simulink model "adaptive"  (R2020a)
settings: Solver=VariableStepAuto  StartTime=0.0  StopTime=30.0  RelTol=1e-3
values from neighbouring files (symbols this model uses):
  Ts = 0.1    [main_adaptive_mpc.m]
libraries: simulink x2, mpclib x1, cstblocks x1
settings Model: Creator=lamarre  LastModifiedBy=Lamarre

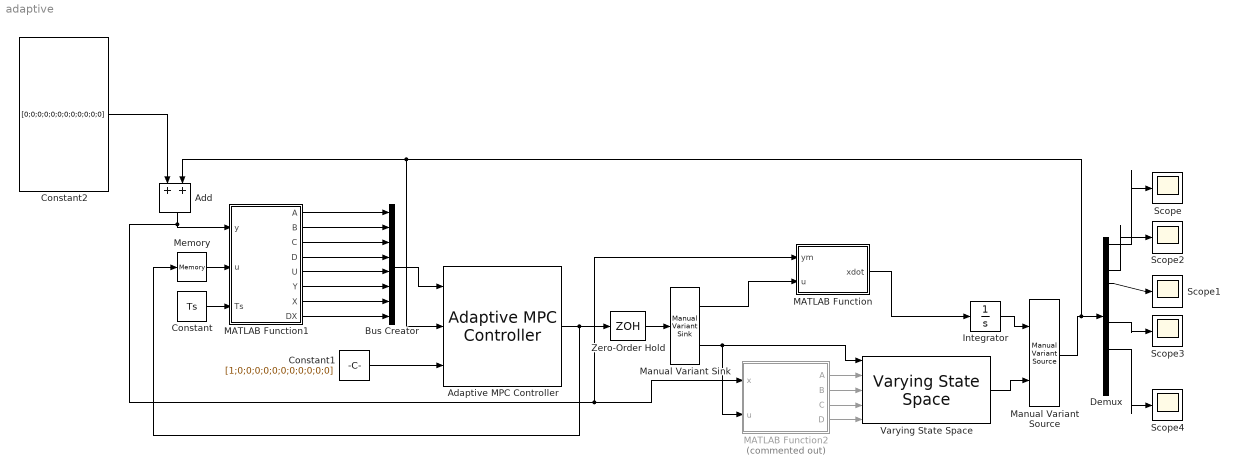
== system adaptive ==
  Adaptive MPC Controller : mpclib/Adaptive MPC Controller  SCDEnableBlockLinearizationSpecification=on  mpcobj=mpcobj  x0=x  enable_value=0  updateMPCinCallerWorkspace=on  md_inport=off  mv_inport=off  uref_inport=off  return_cost=off  return_mvseq=off  return_qpstatus=off  return_xseq=off  return_state=off  return_ovseq=off  state_inport=off  isltv_plant=off  umin_inport=off  umax_inport=off  ymin_inport=off  ymax_inport=off  cc_inport=off  ywt_inport=off  uwt_inport=off  duwt_inport=off  rhoeps_inport=off  pm_inport=off  MaximumP=10  HorizonChoice=FixedHorizon  BlockDataType=double  SampleTimeInherited=off  switch_inport=off
  Add : Sum
  Bus Creator : BusCreator  Inputs=8
  Constant : Constant  Value=Ts
  Constant1 : Constant  Value=[1;0;0;0;0;0;0;0;0;0;0;0]
  Constant2 : Constant  Value=[0;0;0;0;0;0;0;0;0;0;0;0]  VectorParams1D=off
  Demux : Demux  Outputs=12
  Integrator : Integrator
  MATLAB Function : MATLAB Function  TreatAsAtomicUnit=on
  MATLAB Function1 : MATLAB Function  TreatAsAtomicUnit=on
  MATLAB Function2 : MATLAB Function  Commented=on  TreatAsAtomicUnit=on
  Manual Variant Sink : simulink/Signal Routing/Manual Variant Sink  NumChoices=2  LabelModeActiveChoice=V_1
  Manual Variant Source : simulink/Signal Routing/Manual Variant Source  NumChoices=2  LabelModeActiveChoice=V_1
  Memory : Memory
  Scope{,1..4} (5 alike) : Scope
  Varying State Space : cstblocks/Linear Parameter Varying/Varying State Space  x0=0  xNames=''  OutputX=on  OutputDX=on
  Zero-Order Hold : ZeroOrderHold  SampleTime=Ts
  wires:
  Adaptive MPC Controller/1 -> Memory/1, Zero-Order Hold/1
  MATLAB Function/1(xdot) -> Integrator/1
  MATLAB Function1/8(DX) -> Bus Creator/8
  MATLAB Function1/4(D) -> Bus Creator/4
  MATLAB Function1/3(C) -> Bus Creator/3
  MATLAB Function1/2(B) -> Bus Creator/2
  MATLAB Function1/1(A) -> Bus Creator/1
  Constant/1 -> MATLAB Function1/3(Ts)
  Memory/1 -> MATLAB Function1/2(u)
  Constant1/1 -> Adaptive MPC Controller/3
  MATLAB Function1/7(X) -> Bus Creator/7
  MATLAB Function1/6(Y) -> Bus Creator/6
  MATLAB Function1/5(U) -> Bus Creator/5
  Bus Creator/1 -> Adaptive MPC Controller/1
  Constant2/1 -> Add/1
  Add/1 -> MATLAB Function/1(ym), MATLAB Function2/1(x), MATLAB Function1/1(y)
  Demux/1 -> Scope/1
  Demux/4 -> Scope1/1
  Demux/3 -> Scope2/1
  MATLAB Function2/4(D) -> Varying State Space/5
  MATLAB Function2/3(C) -> Varying State Space/4
  MATLAB Function2/2(B) -> Varying State Space/3
  MATLAB Function2/1(A) -> Varying State Space/2
  Zero-Order Hold/1 -> Manual Variant Sink/1
  Manual Variant Sink/2 -> MATLAB Function2/2(u), Varying State Space/1
  Demux/7 -> Scope3/1
  Varying State Space/2 -> Manual Variant Source/2
  Manual Variant Source/1 -> Demux/1, Adaptive MPC Controller/2, Add/2
  Integrator/1 -> Manual Variant Source/1
  Manual Variant Sink/1 -> MATLAB Function/2(u)
  Demux/9 -> Scope4/1

== matlab function adaptive/MATLAB Function1 ==
  data: y input; u input; A output; Ts input; B output; C output; D output; U output; Y output; X output; DX output
function [A,B,C,D,U,Y,X,DX] = Plant(y,u,Ts)
% Lineariser le model dynamique

%x=[y(4:5,1);y(7:12,1)];
%x(5)=x(5)-.85;
[Ac, Bc, Cc, Dc]=AUVStateJacobianFcn(y,u);
% Generate discrete-time model

%  nx = size(Ac,1);
%  nu = size(Bc,2);
%cplant=ss(Ac,Bc,Cc,Dc);
%plant=c2d(cplant,Ts,'zoh');

  M = expm([[Ac Bc]*Ts; zeros(8,16)]);
  A = M(1:8,1:8);
  B = M(1:8,8+1:8+8);
  C = Cc;
 D = Dc;
 %xx=[X(4:5,1);X(7:12)];

% cplant=ss(Ac,Bc,Cc,Dc);
% plant=c2d(cplant,Ts,'zoh');
%plant=ss(A,B,C,D,Ts);

% Nominal conditions for discrete-time plant
U=u.';
Y=(Cc*x + Dc*u).';
X=x.';
DX=(A*x+B*u-x).';

== matlab function adaptive/MATLAB Function ==
  data: ym input; u input; xdot output
function xdot = fcn(ym,u)

xdot = AUVStateFcn(ym,u);

== matlab function adaptive/MATLAB Function2 ==
  data: x input; u input; A output; B output; C output; D output
function [A,B,C,D] = fcn(x,u)
[A B C D]=FullAUVStateJacobianFcn(x,u);
end
